simulink model "function_call_split"  (R2015b)
settings: Solver=VariableStepAuto  StartTime=0.0  StopTime=10.0  RelTol=1e-3
settings Model: Creator=ladmin  LastModifiedBy=ladmin

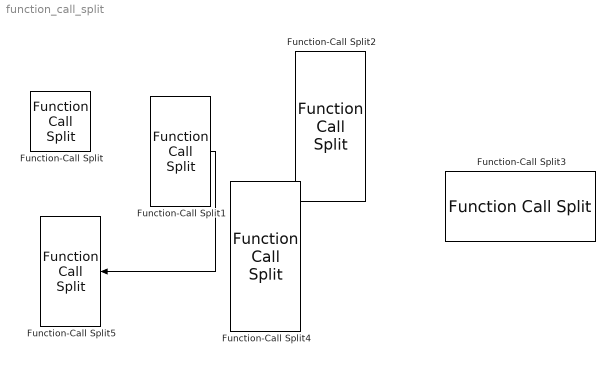
== system function_call_split ==
  Function-Call Split{,1..5} (6 alike) : FunctionCallSplit
  wires:
  Function-Call Split1/1 -> Function-Call Split5/1
